simulink model "SEPIC_PCMC_triangle_compensation"  (R2025a)
settings: Solver=FixedStepAuto  StartTime=0.0  StopTime=1  FixedStep=1e-7  RelTol=1e-3
libraries: spsSeriesRLCBranchLib x5, spsCurrentMeasurementLib x3, spsVoltageMeasurementLib x3, spsGroundLib x2, spsDCVoltageSourceLib x1, spsDiodeLib x1, spsMosfetLib x1, simulink x1, simulink_extras x1, spsVariableResistorLib x1, sps_lib x1
settings Model: Creator=gamezebra  LastModifiedBy=gamezebra

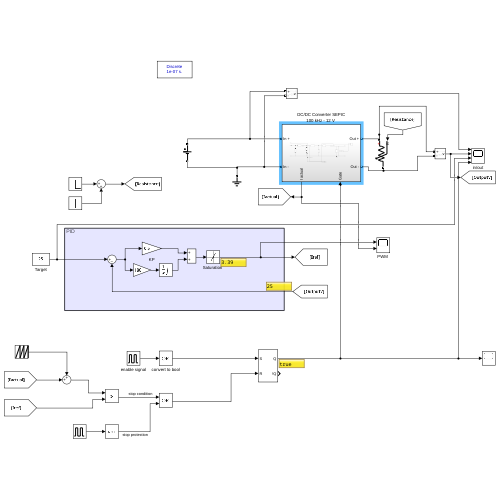
[thumbnail: Simulink's stored preview of the top-level diagram]
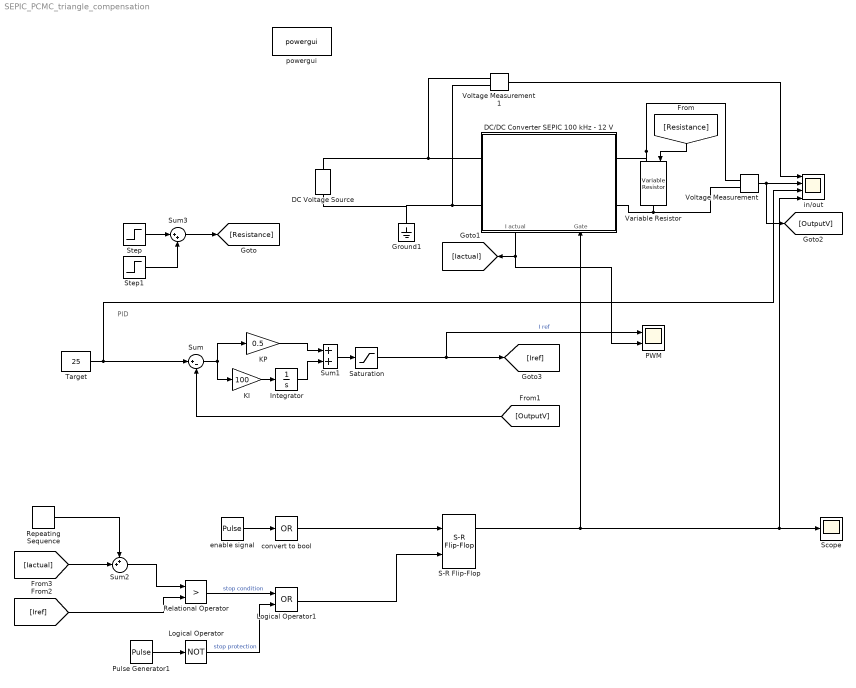
== system SEPIC_PCMC_triangle_compensation ==
  note: PID
  DC Voltage Source : spsDCVoltageSourceLib/DC Voltage Source  Amplitude=16.4  Measurements=None
  "DC/DC Converter SEPIC 100 kHz - 12 V " : Subsystem
      settings: PortSchema="{\"entries\":[{\"content\":{\"sides\":[{\"content\":{\"connectorIds\":[\"LConn1\",\"LConn2\"]},\"type\":\"ConnectorPlacement.EquallySpacedRectSide\",\"uuid\":\"91feb529-5820-4edf-8d0e-1c637fed9421\"},{\"content\":{\"connectorIds\":[\"RConn1\",\"RConn2\"],\"side\":\"RIGHT\"},\"type\":\"ConnectorPlacement.EquallySpacedRectSide\",\"uuid\":\"b4099113-c0ef-4c50-8083-88b14b98cc04\"},{\"content\":{\"side\":\"TOP\"},\"type\":\"ConnectorPlacement.EquallySpacedRectSide\",\"uuid\":\"250c6351-2de3-43d7-b6c9-3c3ed0452184\"},{\"content\":{\"connectorIds\":[\"Out1\",\"In1\"],\"side\":\"BOTTOM\"},\"type\":\"ConnectorPlacement.EquallySpacedRectSide\",\"uuid\":\"484af620-bbf2-4328-991e-a08b15b59058\"}]},\"type\":\"ConnectorPlacement.EquallySpacedConnector\",\"uuid\":\"7041a545-1967-46d5-8643-e26f6c990daf\"}],\"packageUris\":[\"http://schema.mathworks.com/mf0/Connector/R2020b\"],\"version\":\"1.0\"}"
  Ground1 : spsGroundLib/Ground  LConnTagsString=a
  Integrator : Integrator  LimitOutput=on  UpperSaturationLimit=8  LowerSaturationLimit=0
  KI : Gain  Gain=100
  KP : Gain  Gain=0.5
  Logical Operator : Logic  Operator=NOT  AllPortsSameDT=off  OutDataTypeStr=boolean
  Logical Operator1 : Logic  Operator=OR  AllPortsSameDT=off  OutDataTypeStr=boolean
  "PWM " : Scope  NumInputPorts=2
      settings: Title=PWM  ActiveDisplayYMinimum=3.3246670438564179  ActiveDisplayYMaximum=8.2208811739016561  YLabel=Amplitudo
  Pulse Generator1 : DiscretePulseGenerator  PulseType=Time based  Period=10e-6  PulseWidth=90
  Relational Operator : RelationalOperator  Operator=>  OutDataTypeStr=boolean  RndMeth=Simplest  InputSameDT=off
  Repeating Sequence : simulink/Sources/Repeating Sequence  rep_seq_t=[0 10e-6]  rep_seq_y=[0 2]
  S-R Flip-Flop : simulink_extras/Flip Flops/S-R Flip-Flop  initial_condition=0
  "Saturation " : Saturate  UpperLimit=8  LowerLimit=0
  Scope : Scope
      settings: ActiveDisplayYMinimum=-0.12499999999999997  ActiveDisplayYMaximum=1.125  DataLoggingVariableName=ScopeData2
  Step : Step  Time=0.2  Before=50  After=20  SampleTime=0
  Step1 : Step  Time=0.3  After=20  SampleTime=0
  Sum : Sum  Inputs=|+-
  Sum1 : Sum
  Sum2 : Sum  Inputs=++|
  Sum3 : Sum  Inputs=|++
  Target : Constant  Value=25
  Variable Resistor : spsVariableResistorLib/Variable Resistor  Rabsmin=1e-3
      settings: LibrarySourceBlock=sps_lib/Passives/Variable Resistor
  Voltage Measurement : spsVoltageMeasurementLib/Voltage Measurement  PhasorSimulation=off  OutputType=Complex  PSBequivalent=0
  Voltage Measurement1 : spsVoltageMeasurementLib/Voltage Measurement  PhasorSimulation=off  OutputType=Complex  PSBequivalent=0
  convert to bool : Logic  Operator=OR  Inputs=1  AllPortsSameDT=off  OutDataTypeStr=boolean
  enable signal : DiscretePulseGenerator  PulseType=Time based  Period=10e-6  PulseWidth=5
  in/out : Scope  NumInputPorts=4
      settings: Title=PWM  ActiveDisplayYMinimum=-3.419102957211801  ActiveDisplayYMaximum=30.741030708134929  YLabel=Amplitudo  DataLoggingVariableName=ScopeData3
  powergui : sps_lib/powergui  Priority=1  SimulationMode=Discrete  SampleTime=1e-7  frequency=60  Iterations=50  frequencyindice=0  Pbase=100e6  ErrMax=1e-4  UnitsV=kV  UnitsW=MW  buscounter=0  FunctionMessages=off  echomessages=off  EnableUseOfTLC=off  CurrentSourceSwitches=off  DisableSnubberDevices=off  DisableRonSwitches=off  DisableVfSwitches=off  DisplayEquations=off  AutomaticDiscreteSolvers=off  SolverType=Tustin/Backward Euler (TBE)  Interpol=off  ExternalGateDelay=off  methode=off  Ts=100  x0status=blocks  SPID=on  SwTol=0  HookPort=off  NonlinearTolerance=1e-4  nMaxIteration=100  ContinueOnMaxIteration=off  RestoreLinks=warning  ResistiveCurrentMeasurement=off  Frange=[0:2:500]  Ylog=off  Xlog=on  ShowGrid=off  save=off  variable=ZData  structure=0  ZoomFFT=off  StartTime=0.0  cycles=1  DisplayStyle=1  fundamental=60  FreqAxis=off  MaxFrequency=1000  frequencyindicesteady=1  RmsSteady=1  display=off
  wires:
  Voltage Measurement1/1 -> in/out/1
  Voltage Measurement/1 -> [OutputV], in/out/2
  [Resistance] -> Variable Resistor/1
  Step/1 -> Sum3/1
  Target/1 -> in/out/3, Sum/1
  Sum1/1 -> "Saturation "/1
  KI/1 -> Integrator/1
  Integrator/1 -> Sum1/2
  KP/1 -> Sum1/1
  Sum/1 -> KI/1, KP/1
  "Saturation "/1 -> "PWM "/1, [Iref]  "I ref"
  [OutputV] -> Sum/2
  S-R Flip-Flop/1 -> in/out/4, Scope/1, "DC/DC Converter SEPIC 100 kHz - 12 V "/1(Gate)
  [Iactual] -> Sum2/2
  Pulse Generator1/1 -> Logical Operator/1
  Relational Operator/1 -> Logical Operator1/1  "stop condition"
  Logical Operator/1 -> Logical Operator1/2  "stop protection"
  "DC/DC Converter SEPIC 100 kHz - 12 V "/1(I actual) -> "PWM "/2, [Iactual]
  [Iref] -> Relational Operator/2
  Logical Operator1/1 -> S-R Flip-Flop/2
  enable signal/1 -> convert to bool/1
  convert to bool/1 -> S-R Flip-Flop/1
  Repeating Sequence/1 -> Sum2/1
  Sum2/1 -> Relational Operator/1
  Step1/1 -> Sum3/2
  Sum3/1 -> [Resistance]
  connections:
  Voltage Measurement1/LConn1 -- DC Voltage Source/RConn1 -- "DC/DC Converter SEPIC 100 kHz - 12 V "/LConn1
  "DC/DC Converter SEPIC 100 kHz - 12 V "/RConn1 -- Voltage Measurement/LConn1 -- Variable Resistor/LConn1
  "DC/DC Converter SEPIC 100 kHz - 12 V "/RConn2 -- Voltage Measurement/LConn2 -- Variable Resistor/RConn1
  "DC/DC Converter SEPIC 100 kHz - 12 V "/LConn2 -- Voltage Measurement1/LConn2 -- DC Voltage Source/LConn1 -- Ground1/LConn1

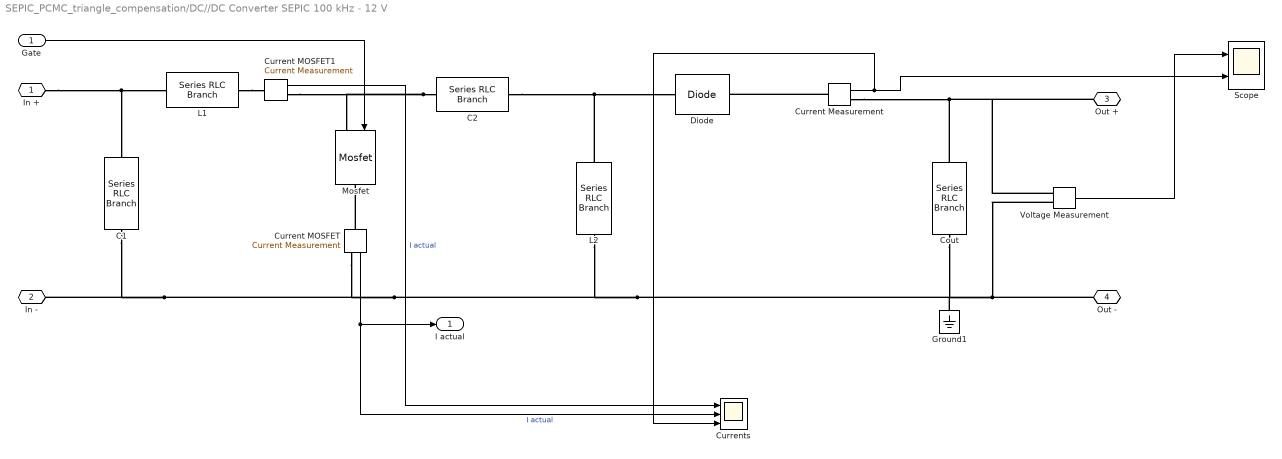
== system SEPIC_PCMC_triangle_compensation/DC//DC Converter SEPIC 100 kHz - 12 V  ==
  Gate : Inport
  C1 : spsSeriesRLCBranchLib/Series RLC Branch  LConnTagsString=__new0  RConnTagsString=__new0  BranchType=RC  Resistance=0.01  Inductance=1e-3  SetiL0=off  InitialCurrent=0  Capacitance=0.0001  Setx0=off  InitialVoltage=0  Measurements=None
  C2 : spsSeriesRLCBranchLib/Series RLC Branch  LConnTagsString=__new0  RConnTagsString=__new0  BranchType=C  Resistance=1  Inductance=1e-3  SetiL0=off  InitialCurrent=0  Capacitance=0.00001  Setx0=off  InitialVoltage=0  Measurements=None
  Cout : spsSeriesRLCBranchLib/Series RLC Branch  LConnTagsString=__new0  RConnTagsString=__new0  BranchType=RC  Resistance=0.01  Inductance=16.8e-3  SetiL0=off  InitialCurrent=0  Capacitance=0.0001  Setx0=off  InitialVoltage=0  Measurements=None
  Current MOSFET : spsCurrentMeasurementLib/Current Measurement  PhasorSimulation=off  OutputType=Complex  PSBequivalent=0
  Current MOSFET1 : spsCurrentMeasurementLib/Current Measurement  PhasorSimulation=off  OutputType=Complex  PSBequivalent=0
  "Current Measurement " : spsCurrentMeasurementLib/Current Measurement  PhasorSimulation=off  OutputType=Complex  PSBequivalent=0
  Currents : Scope  NumInputPorts=3
      settings: ActiveDisplayYMinimum=-0.85479066123775027  ActiveDisplayYMaximum=4.4139964781380261  DataLoggingVariableName=ScopeData4
  "Diode " : spsDiodeLib/Diode  Ron=0.001  Lon=0  Vf=0.5  IC=0  UseSnubber=0  Rs=500  Cs=250e-9  Measurements=off
  Ground1 : spsGroundLib/Ground  LConnTagsString=a
  L1 : spsSeriesRLCBranchLib/Series RLC Branch  LConnTagsString=__new0  RConnTagsString=__new0  BranchType=RL  Resistance=0.2  Inductance=0.0002  SetiL0=off  InitialCurrent=0  Capacitance=1e-6  Setx0=off  InitialVoltage=0  Measurements=None
  L2 : spsSeriesRLCBranchLib/Series RLC Branch  LConnTagsString=__new0  RConnTagsString=__new0  BranchType=RL  Resistance=0.2  Inductance=0.0002  SetiL0=off  InitialCurrent=0  Capacitance=1e-6  Setx0=off  InitialVoltage=0  Measurements=None
  Mosfet : spsMosfetLib/Mosfet  Ron=0.1  Lon=0  Rd=0.01  Vfd=0  IC=0  Rs=1e5  Cs=inf  Measurements=off
  Scope : Scope  NumInputPorts=2
      settings: Title=Tegangan Keluaran Konverter SEPIC  ActiveDisplayYMinimum=-151.86738214367281  ActiveDisplayYMaximum=1366.8064463408562  YLabel=Tegangan (Volts)
  "Voltage Measurement " : spsVoltageMeasurementLib/Voltage Measurement  PhasorSimulation=off  OutputType=Complex  PSBequivalent=0
  In + : PMIOPort  Side=Left
  In - : PMIOPort  Port=2  Side=Left
  Out + : PMIOPort  Port=3  Side=Right
  Out - : PMIOPort  Port=4  Side=Right
  I actual : Outport
  wires:
  Gate/1 -> Mosfet/1
  "Current Measurement "/1 -> Currents/3, Scope/2
  "Voltage Measurement "/1 -> Scope/1
  Current MOSFET/1 -> Currents/2, I actual/1  "I actual"
  Current MOSFET1/1 -> Currents/1  "I actual"
  connections:
  Out -/RConn1 -- Cout/RConn1 -- Ground1/LConn1 -- L2/RConn1 -- C1/RConn1 -- In -/RConn1 -- Current MOSFET/RConn1 -- "Voltage Measurement "/LConn2
  C2/LConn1 -- Current MOSFET1/RConn1 -- Mosfet/LConn1
  C2/RConn1 -- L2/LConn1 -- "Diode "/LConn1
  Cout/LConn1 -- "Voltage Measurement "/LConn1 -- Out +/RConn1 -- "Current Measurement "/RConn1
  In +/RConn1 -- C1/LConn1 -- L1/LConn1
  "Current Measurement "/LConn1 -- "Diode "/RConn1
  Current MOSFET/LConn1 -- Mosfet/RConn1
  L1/RConn1 -- Current MOSFET1/LConn1
